simulink model "HF_simulink"  (R2018b)
settings: Solver=VariableStepAuto  StartTime=0.0  StopTime=30  RelTol=1e-3
undefined symbols (not defined in the file): g, Iyy, l1, m
libraries: vrlib x3
settings Model: Creator=ferra  LastModifiedBy=ferra

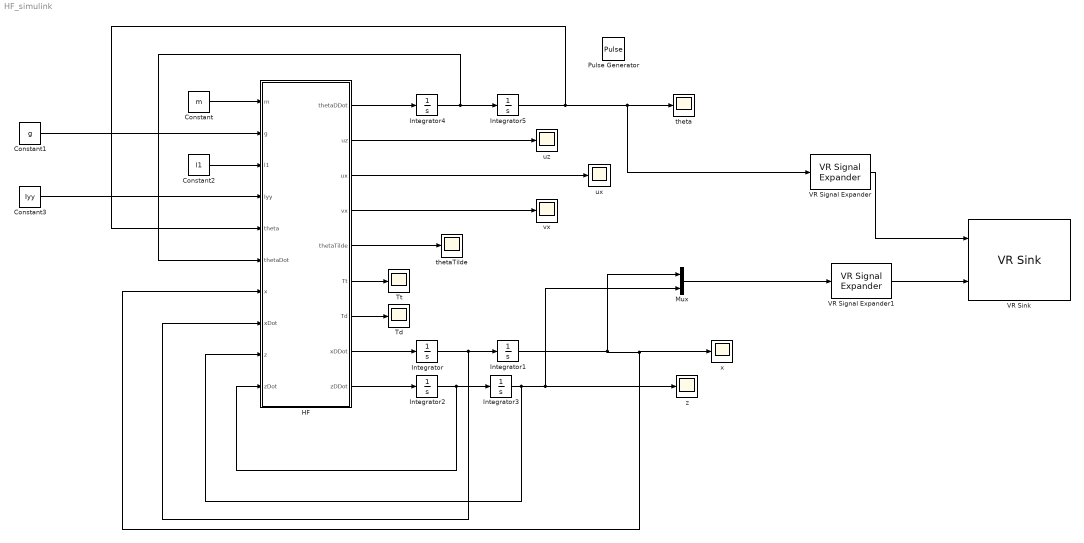
== system HF_simulink ==
  Constant : Constant  Value=m
  Constant1 : Constant  Value=g
  Constant2 : Constant  Value=l1
  Constant3 : Constant  Value=Iyy
  "HF " : MATLAB Function  TreatAsAtomicUnit=on
  Integrator{,1..2,4} (4 alike) : Integrator
  Integrator3 : Integrator  InitialCondition=-3
  Integrator5 : Integrator  InitialCondition=pi/8
  Mux : Mux  Inputs=2
  Pulse Generator : DiscretePulseGenerator  PulseType=Time based  Amplitude=pi/8  Period=15  PulseWidth=5
  Td : Scope
  Tt : Scope
  VR Signal Expander : vrlib/VR Signal Expander  outwidth=4  outidx=[4]
      settings: SourceProductName=Simulink 3D Animation  SourceProductBaseCode=VR
  VR Signal Expander1 : vrlib/VR Signal Expander  outwidth=3  outidx=[1 2]
      settings: SourceProductName=Simulink 3D Animation  SourceProductBaseCode=VR
  VR Sink : vrlib/VR Sink  InstantiateOnLoad=on  SampleTime=0.1  ViewEnable=on  RemoteChange=off  RemoteView=off  FieldsWritten=Airplane.rotation.4.1.1.double#Airplane.translation.3.1.1.double  WorldFileName=C:\Users\ferra\Desktop\Projects\Matlab\Thesis\3D-simulation\HF_3d.WRL  AutoView=off  VideoDimensions=[]  AllowVariableSize=off
      settings: SourceProductBaseCode=VR
  theta : Scope
  thetaTilde : Scope
  ux : Scope
  uz : Scope
  vx : Scope
  x : Scope
  z : Scope
  wires:
  "HF "/6(Tt) -> Tt/1
  "HF "/3(ux) -> ux/1
  Integrator5/1 -> "HF "/5(theta), VR Signal Expander/1, theta/1
  Integrator3/1 -> Mux/2, z/1, "HF "/9(z)
  Constant1/1 -> "HF "/2(g)
  "HF "/5(thetaTilde) -> thetaTilde/1
  Integrator1/1 -> x/1, "HF "/7(x), Mux/1
  "HF "/2(uz) -> uz/1
  Constant/1 -> "HF "/1(m)
  Constant2/1 -> "HF "/3(l1)
  Integrator4/1 -> "HF "/6(thetaDot), Integrator5/1
  "HF "/1(thetaDDot) -> Integrator4/1
  "HF "/9(zDDot) -> Integrator2/1
  Integrator/1 -> Integrator1/1, "HF "/8(xDot)
  Constant3/1 -> "HF "/4(Iyy)
  Integrator2/1 -> Integrator3/1, "HF "/10(zDot)
  "HF "/7(Td) -> Td/1
  "HF "/8(xDDot) -> Integrator/1
  "HF "/4(vx) -> vx/1
  VR Signal Expander/1 -> VR Sink/1
  Mux/1 -> VR Signal Expander1/1
  VR Signal Expander1/1 -> VR Sink/2

== matlab function HF_simulink/HF  ==
  data: thetaDDot output; uz output; ux output; vx output; thetaTilde output; Tt output; Td output; m input; xDDot output; g input; l1 input; Iyy input; theta input; thetaDot input; x input; xDot input; z input; zDot input; zDDot output
function [thetaDDot,uz,ux,vx,thetaTilde,Tt,Td,xDDot,zDDot] = HF_dynamics(m,g,l1,Iyy,theta,thetaDot,x,xDot,z,zDot)

kpz = 7;
kdz = 5;
kpx = 5;
kdx = 15;

zDes = 3;
xDes = 4;
eX = x-xDes;
%virtual controllers
uz = -kpz*(z-zDes) - kdz * zDot; 
vx = -kpx*(eX) - kdx * xDot;
ux = atan(vx/(uz-g));

%error
thetaTilde = theta - ux;


Tt = -(m*uz - m*g)/(cos(theta));

Td = (tanh(thetaTilde) + tanh(thetaDot))/(l1);

xDDot = -Tt * sin(theta)/m;
zDDot = -Tt * cos(theta)/m + g;
thetaDDot = -Td*l1/Iyy;

end
